simulink model "ZeroOrderHoldFunctionTest"  (Simulink 7.7)
settings: Solver=VariableStepDiscrete  StartTime=0.0  StopTime=0.25  RelTol=1e-3
values from neighbouring files (symbols this model uses):
  L = Fsam*10    (= 10000)    [BPSK_selfmade.m]    (also in DAC_fft.m = 2000; InterpolateSignalVector.m = 1024; TP_BP_Spektrum.m = length(t); fft_whyFactorL.m = 1000)
  Ts = Tsam*Fsam    (= 1)    [BPSK_selfmade.m]    (also in FFT_iFFT.m = 0.0002; InterpolateSignalVector.m = 0.0025; QPSK_constellation.m; correlationSample.m)
undefined symbols (not defined in the file or in its folder): f1Dac
libraries: simulink_extras x1, simulink x1
settings Model: Creator=mainster  LastModifiedBy=mainster

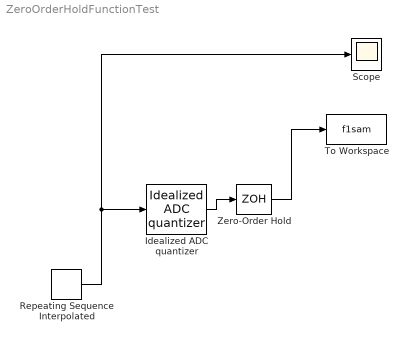
== system ZeroOrderHoldFunctionTest ==
  Idealized ADC quantizer : simulink_extras/Additional Discrete/Idealized ADC quantizer  SystemSampleTime=-1  NumberOfConverterBits=12  Vmin=-1  Vmax=1  OutputDataType=int16  OutputNegativeValues=on
  Repeating Sequence Interpolated : simulink/Sources/Repeating Sequence Interpolated  SystemSampleTime=-1  OutValues=f1Dac(L/2+1:L-1)  TimeValues=t(L/2+1:L-1)  LookUpMeth=Interpolation-Use End Values  tsamp=Ts  OutMin=[]  OutMax=[]  OutDataTypeStr=double  OutputDataTypeScalingMode=double  OutDataType=fixdt(0,8)  OutScaling=2^-10
  Scope : Scope
  To Workspace : ToWorkspace  VariableName=f1sam  SampleTime=-1  SaveFormat=Structure
  Zero-Order Hold : ZeroOrderHold  SampleTime=Ts*3
  wires:
  Repeating Sequence Interpolated/1 -> Idealized ADC quantizer/1, Scope/1
  Idealized ADC quantizer/1 -> Zero-Order Hold/1
  Zero-Order Hold/1 -> To Workspace/1
